simulink subsystem "Subsystem_EncoderVelocidad"  (R2023b)
settings: Solver=VariableStepAuto  StartTime=0.0  StopTime=10.0  RelTol=1e-3
libraries: arduinosensorlib x2, simulink x1
settings Model: Creator=Alberto  LastModifiedBy=Alberto

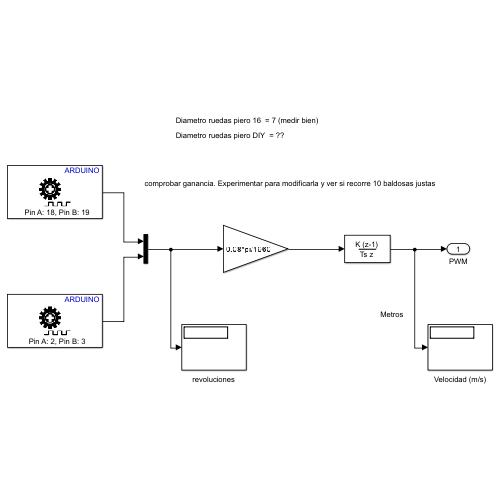
[thumbnail: Simulink's stored preview of the top-level diagram]
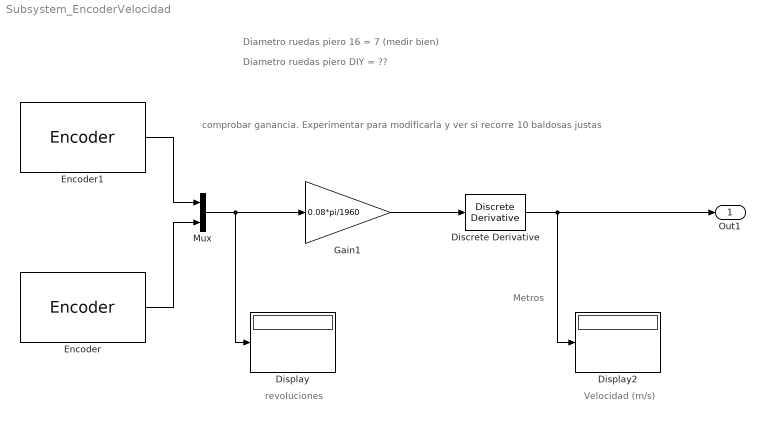
== system Subsystem_EncoderVelocidad ==
  note: revoluciones
  note: Velocidad (m/s)
  note: Metros
  note: comprobar ganancia. Experimentar para modificarla y ver si recorre 10 baldosas justas
  note: Diametro ruedas piero 16 = 7 (medir bien)
  note: Diametro ruedas piero DIY = ??
  Discrete Derivative : simulink/Discrete/Discrete Derivative  gainval=1.0  ICPrevScaledInput=0.0  OutMin=[]  OutMax=[]  OutDataType=fixdt(1, 16)  OutScaling=2^-10  DoSatur=off
  Display : Display
  Display2 : Display
  Encoder : arduinosensorlib/Encoder  InputA=2  InputB=3  Mode=No reset  SampleTime=-1
  Encoder1 : arduinosensorlib/Encoder  InputA=18  InputB=19  Mode=No reset  SampleTime=-1
  Gain1 : Gain  Gain=0.08*pi/1960
  Mux : Mux  Inputs=2
  Out1 : Outport
  wires:
  Mux/1 -> Gain1/1, Display/1
  Gain1/1 -> Discrete Derivative/1
  Encoder1/1 -> Mux/1
  Encoder/1 -> Mux/2
  Discrete Derivative/1 -> Display2/1, Out1/1
